simulink model "Final_Model_3"  (R2022a)
settings: Solver=VariableStepAuto  StartTime=0.0  StopTime=30  MaxStep=0.01  RelTol=1e-3
values from neighbouring files (symbols this model uses):
  Kb = p.Kb    [noise_step.m]    (also in pid_step.m; sensitivity.m; td_sim.m; torquesim.m)
  Kd = p.Kd    [noise_step.m]    (also in sensitivity.m; td_sim.m; torquesim.m)
  Ki = p.Ki    [noise_step.m]    (also in sensitivity.m; td_sim.m; torquesim.m)
  Km = p.Km    [noise_step.m]    (also in pid_step.m; sensitivity.m; td_sim.m; torquesim.m)
  Kp = p.Kp    [noise_step.m]    (also in sensitivity.m; td_sim.m; torquesim.m)
  N = p.N    [noise_step.m]    (also in pid_step.m; sensitivity.m; td_sim.m; torquesim.m)
  Ra = p.Ra    [noise_step.m]    (also in pid_step.m; sensitivity.m; td_sim.m; torquesim.m)
undefined symbols (not defined in the file or in its folder): config
libraries: simulink x1, cstblocks x1
settings Model: Creator=natha  LastModifiedBy=natha
settings SolverCC: MaxConsecutiveMinStep=2
settings DataIOCC: SaveFormat=StructureWithTime  InspectSignalLogs=on
settings OptimizationCC: GainParamInheritBuiltInType=on
settings ModelReferenceCC: EnableParallelModelReferenceBuilds=on  ParallelModelReferenceMATLABWorkerInit=Copy Base Workspace
settings SFSimCC: SimTargetLang=C++  GPUAcceleration=on  SimDLTargetLibrary=cudnn

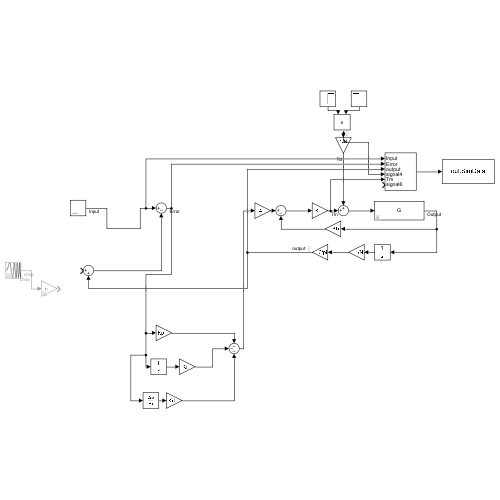
[thumbnail: Simulink's stored preview of the top-level diagram]
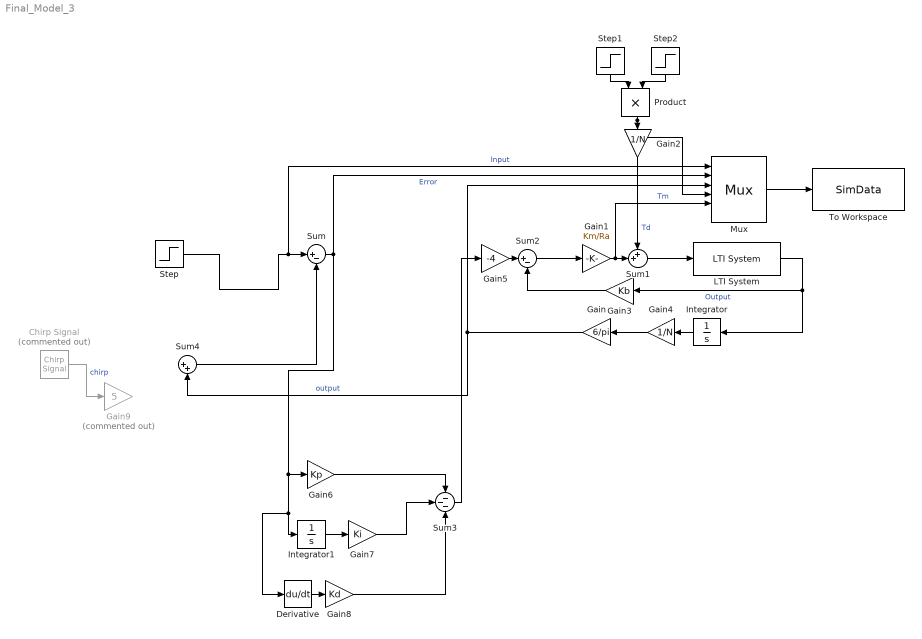
== system Final_Model_3 ==
  Chirp Signal : simulink/Sources/Chirp Signal  Commented=on  f1=30000  T=100  f2=100000
  Derivative : Derivative
  Gain : Gain  Gain=6/pi
  Gain1 : Gain  Gain=Km/Ra
  Gain2 : Gain  Gain=1/N
  Gain3 : Gain  Gain=Kb
  Gain4 : Gain  Gain=1/N
  Gain5 : Gain  Gain=-4
  Gain6 : Gain  Gain=Kp
  Gain7 : Gain  Gain=Ki
  Gain8 : Gain  Gain=Kd
  Gain9 : Gain  Commented=on  Gain=5
  Integrator : Integrator
  Integrator1 : Integrator
  LTI System : cstblocks/LTI System  sys=G  IC=[]
  Mux : Mux  Inputs=6
      settings: DisplayOption=signals
  Product : Product
  Step : Step  Time=config.stepTime  After=config.stepSize  SampleTime=0
  Step1 : Step  Time=config.torqueStart  After=config.Td  SampleTime=0
  Step2 : Step  Time=config.torqueEnd  Before=1  After=0  SampleTime=0
  Sum : Sum  Inputs=|+-
  Sum1 : Sum  Inputs=++|
  Sum2 : Sum  Inputs=|+-
  Sum3 : Sum  Inputs=---
  Sum4 : Sum  Inputs=|++
  To Workspace : ToWorkspace  VariableName=SimData  SaveFormat=Structure With Time  SampleTime=-1
  wires:
  Sum/1 -> Derivative/1, Integrator1/1, Gain6/1, Mux/2  "Error"
  Mux/1 -> To Workspace/1
  Gain/1 -> Sum4/2, Mux/3  "output"
  Gain1/1 -> Mux/5, Sum1/2  "Tm"
  Gain2/1 -> Sum1/1  "Td"
  Step2/1 -> Product/2
  Step1/1 -> Product/1
  Product/1 -> Mux/4, Gain2/1
  Gain3/1 -> Sum2/2
  Integrator/1 -> Gain4/1
  Gain4/1 -> Gain/1
  LTI System/1 -> Gain3/1, Integrator/1  "Output"
  Sum1/1 -> LTI System/1
  Gain5/1 -> Sum2/1
  Sum2/1 -> Gain1/1
  Gain6/1 -> Sum3/1
  Gain8/1 -> Sum3/3
  Step/1 -> Mux/1, Sum/1  "Input"
  Integrator1/1 -> Gain7/1
  Derivative/1 -> Gain8/1
  Gain7/1 -> Sum3/2
  Sum3/1 -> Gain5/1
  Sum4/1 -> Sum/2
  Chirp Signal/1 -> Gain9/1  "chirp"
